simulink model "AD_Snowman"  (R2023b)
settings: Solver=FixedStepDiscrete  StartTime=0.0  StopTime=1  FixedStep=0.01  RelTol=1e-3
StopFcn:
  | Copy_of_AD_Display_Plot;
libraries: AD_Snowman_Library x5, simulink x1
settings Model: LastModifiedBy=ander

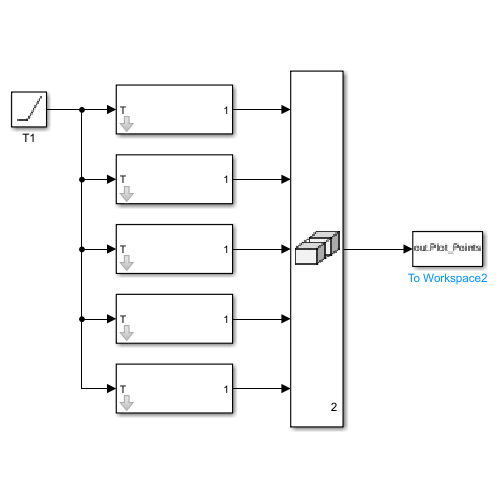
[thumbnail: Simulink's stored preview of the top-level diagram]
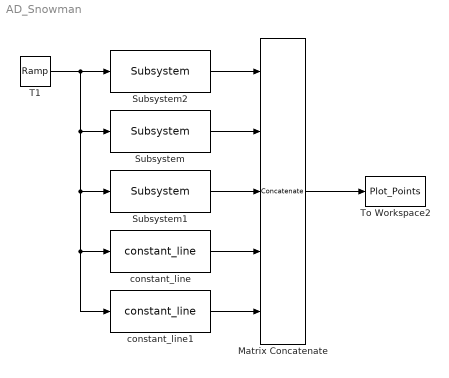
== system AD_Snowman ==
  Matrix Concatenate : Concatenate  NumInputs=5  Mode=Multidimensional array  ConcatenateDimension=2
  Subsystem : AD_Snowman_Library/Subsystem  X_Offset=2  Y_Offset=4  A=1  B=1
  Subsystem1 : AD_Snowman_Library/Subsystem  X_Offset=2  Y_Offset=1  A=2  B=2
  Subsystem2 : AD_Snowman_Library/Subsystem  X_Offset=2  Y_Offset=5.5  A=0.5  B=0.5
  T1 : simulink/Sources/Ramp  slope=1  start=0  InitialOutput=0
  To Workspace2 : ToWorkspace  VariableName=Plot_Points  SampleTime=-1
  constant_line : AD_Snowman_Library/constant_line  P0=[4 1]  P1=[5 -1]
  constant_line1 : AD_Snowman_Library/constant_line  P0=[4 3]  P1=[5 5]
  wires:
  Matrix Concatenate/1 -> To Workspace2/1
  Subsystem1/1 -> Matrix Concatenate/3
  Subsystem/1 -> Matrix Concatenate/2
  Subsystem2/1 -> Matrix Concatenate/1
  T1/1 -> Subsystem/1, constant_line1/1, constant_line/1, Subsystem1/1, Subsystem2/1
  constant_line/1 -> Matrix Concatenate/4
  constant_line1/1 -> Matrix Concatenate/5
